simulink model "schema"  (R2021b)
settings: Solver=VariableStepAuto  StartTime=0.0  StopTime=20.0  RelTol=1e-3
undefined symbols (not defined in the file): k, wn, xi
settings Model: Creator=User  LastModifiedBy=User

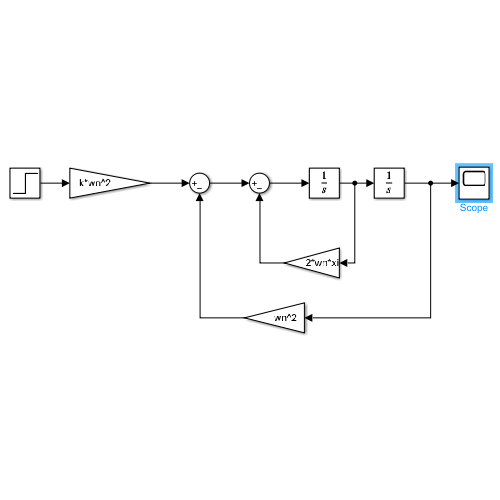
[thumbnail: Simulink's stored preview of the top-level diagram]
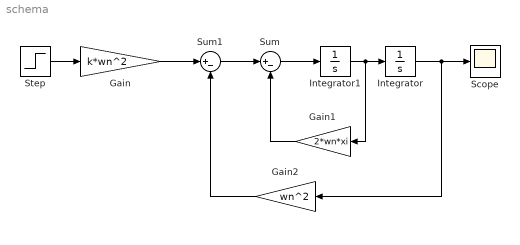
== system schema ==
  Gain : Gain  Gain=k*wn^2
  Gain1 : Gain  Gain=2*wn*xi
  Gain2 : Gain  Gain=wn^2
  Integrator : Integrator
  Integrator1 : Integrator
  Scope : Scope
  Step : Step  SampleTime=0
  Sum : Sum  Inputs=|+-
  Sum1 : Sum  Inputs=|+-
  wires:
  Sum1/1 -> Sum/1
  Gain/1 -> Sum1/1
  Sum/1 -> Integrator1/1
  Integrator1/1 -> Gain1/1, Integrator/1
  Step/1 -> Gain/1
  Integrator/1 -> Gain2/1, Scope/1
  Gain2/1 -> Sum1/2
  Gain1/1 -> Sum/2
